simulink model "generic_IVS"  (R2024a)
settings: Solver=FixedStepDiscrete  StartTime=0.0  StopTime=inf  FixedStep=0.001  RelTol=1e-3
undefined symbols (not defined in the file): do_waypoints_tail_shifted_2, pathXY, route1_waypoint, route1_waypoint_raw, route2_waypoint, route2_waypoint_raw, route3_waypoint, route3_waypoint_raw, waypoints2
libraries: CarMaker4SL x431, slpidlib x19, dspsigops x3, simulink x1
(part 12 of 15)

== matlab function generic_IVS/CarMaker/Subsystem/Final Project1/Scenario 1/Enabled Subsystem2/MATLAB Function3 ==
  settings: updateMethod=DISCRETE  sampleTime=0.05
  data: map_boundary input; mapMatrix output size=[1000, 1000]; traffic_info input
%% ======== generate_map_ ======== Ver 2025-05-17 10:40
function mapMatrix  = generate_map_(map_boundary, traffic_info)
    %변수설정
    resolution = 0.05;
    traffic_info_mat = reshape(traffic_info(1:5*21), 5, []).';
    x_values = map_boundary(1:2:end);
    y_values = map_boundary(2:2:end);
    N = size(traffic_info_mat,1);
    x_min = min(x_values);  x_max = max(x_values);
    y_min = min(y_values);  y_max = max(y_values);
    x_size = ceil((x_max-x_min)/resolution);
    y_size = ceil((y_max-y_min)/resolution);
    
    
    mapMatrix = zeros(y_size, x_size); %출력코드
    
    for i = 1:N
        x_c = traffic_info_mat(i, 1);
        y_c = traffic_info_mat(i, 2);
        yaw = traffic_info_mat(i, 3);
        length = traffic_info_mat(i, 4);
        width = traffic_info_mat(i, 5);
        
        if yaw == -1.57079628
            yaw = -pi/2;
        elseif yaw == 1.57079628
            yaw = pi/2;
        end

        dx = length/2;  dy = width/2;
        local = [-dx,-dy; dx,-dy; dx,dy; -dx,dy];
        R = [cos(yaw), -sin(yaw); sin(yaw), cos(yaw)];
        rotated = (R*local')';
        forward_vec = [cos(yaw), sin(yaw)];
        side_vec    = [-sin(yaw), cos(yaw)];
        if yaw == -pi/2
            center = [x_c, y_c] + (length/2)*forward_vec + (width/2)*side_vec;
        else
            center = [x_c, y_c] + (length/2)*forward_vec - (width/2)*side_vec;
        end
        corners = rotated + center;
        x_idx = (corners(:,1)-x_min)/resolution + 1;
        y_idx = (y_max-corners(:,2))/resolution + 1;
        mask = poly2mask(x_idx, y_idx, y_size, x_size);
        mapMatrix(mask) = 1;
    end
end

== matlab function generic_IVS/CarMaker/Subsystem/Final Project1/Scenario 1/Enabled Subsystem2/MATLAB Function4 ==
  settings: updateMethod=DISCRETE  sampleTime=0.05
  data: map input; x_path output; startPose input; goalPose input; y_path output; mapboundary input
function [x_path, y_path] = rrt_star_planner(map, startPose, goalPose, mapboundary)
    %% ===== Persistent 저장 =====
    persistent path_initialized x_path_cached y_path_cached nPath_cached
    maxPathLength = 500;
    resolution = 0.05;

    if isempty(path_initialized)
        path_initialized = false;
        x_path_cached = zeros(maxPathLength, 1);
        y_path_cached = zeros(maxPathLength, 1);
        nPath_cached = 1;
    end

    if path_initialized
        x_path = x_path_cached(1:nPath_cached);
        y_path = y_path_cached(1:nPath_cached);
        return;
    end

    %% 설정
    visualize      = false;
    maxIter        = 5000;
    stepSize       = 2;
    goalSampleRate = 0.1;
    successDistTh  = 5;
    collisionRes   = 0.5;
    searchRadius   = 10;
    safetyDist     = 35;
    
    %% 바운더리 기반 인덱스 변환용 파라미터
    x_values = mapboundary(1:2:end);
    y_values = mapboundary(2:2:end);
    x_min = min(x_values);
    y_max = max(y_values);

    %% 실좌표 → 인덱스 변환
    toGrid = @(x, y) [(x - x_min)/resolution +  1, (y_max - y)/resolution + 1];

    start_grid = toGrid(startPose(1), startPose(2));
    goal_grid  = toGrid(goalPose(1), goalPose(2));

    %% 트리 초기화 (모든 노드는 인덱스 좌표로 유지)
    nodes = struct('x', start_grid(1), 'y', start_grid(2), ...
                   'parent', 0, 'cost', 0);

    %% 경로 및 출력 초기화
    path   = struct('x', {}, 'y', {}, 'parent', {}, 'cost', {});
    x_path = zeros(maxPathLength, 1);
    y_path = zeros(maxPathLength, 1);

    %% RRT* 메인 루프 (모든 연산 인덱스 기반)
    for iter = 1:maxIter
        if rand < goalSampleRate
            xr = goal_grid;
        else
            xr = [randi([1, size(map,2)]), randi([1, size(map,1)])];
        end

        [nearestIdx, nearXY] = findNearest(nodes, xr);
        theta = atan2(xr(2)-nearXY(2), xr(1)-nearXY(1));
        newXY = nearXY + stepSize * [cos(theta), sin(theta)];

        if isCollision(newXY, map) || ...
           isPathCollision(nearXY, newXY, map, collisionRes) || ...
           isNearObstacle(newXY, map, safetyDist)
            continue;
        end

        nearIdxs = findNearNodes(nodes, newXY, searchRadius);
        minCost   = nodes(nearestIdx).cost + norm(newXY - nearXY);
        minParent = nearestIdx;

        for idx = 1:numel(nearIdxs)
            iNode = nearIdxs(idx);
            pxy   = [nodes(iNode).x, nodes(iNode).y];
            if ~isPathCollision(pxy, newXY, map, collisionRes)
                c = nodes(iNode).cost + norm(newXY - pxy);
                if c < minCost
                    minCost   = c;
                    minParent = iNode;
                end
            end
        end

        newNode = struct('x', newXY(1), 'y', newXY(2), ...
                         'parent', minParent, 'cost', minCost);
        nodes(end+1) = newNode;
        newIdx       = numel(nodes);

        for idx = 1:numel(nearIdxs)
            iNode = nearIdxs(idx);
            pxy   = [nodes(iNode).x, nodes(iNode).y];
            c     = newNode.cost + norm([newNode.x, newNode.y] - pxy);
            if c < nodes(iNode).cost && ...
               ~isPathCollision([newNode.x,newNode.y], pxy, map, collisionRes)
                nodes(iNode).parent = newIdx;
                nodes(iNode).cost   = c;
            end
        end

        if visualize
            plot([nodes(newNode.parent).x, newNode.x], ...
                 [nodes(newNode.parent).y, newNode.y], '-r');
            hold on;
        end

        if norm(newXY - goal_grid) < successDistTh
            if visualize, disp('[-] GOAL REACHED'); end
            path = backtrace(nodes, newIdx);
            break;
        end
    end

    %% 결과 경로 반환 (인덱스 → 실좌표로 역변환)
    nPath = min(numel(path), maxPathLength);
    x_path_cached = zeros(maxPathLength, 1);
    y_path_cached = zeros(maxPathLength, 1);
    for k = 1:nPath
        x_path_cached(k) = (path(k).x - 1) * resolution + x_min;
        y_path_cached(k) = y_max - (path(k).y - 1) * resolution;
    end

    nPath_cached = nPath;
    path_initialized = true;

    %% === Lightweight Smoothing for Simulink Compatibility ===
    smooth_window = 15;  % 홀수 추천
    if nPath >= smooth_window
        x = x_path_cached(1:nPath);
        y = y_path_cached(1:nPath);

        x_smooth = movmean(x, smooth_window);
        y_smooth = movmean(y, smooth_window);

        % 재샘플링 (고정된 개수로)
        smoothN = 100;
        idx_original = linspace(1, numel(x_smooth), smoothN);
        x_path = interp1(1:numel(x_smooth), x_smooth, idx_original, 'linear')';
        y_path = interp1(1:numel(y_smooth), y_smooth, idx_original, 'linear')';
    else
        x_path = x_path_cached(1:nPath);
        y_path = y_path_cached(1:nPath);
    end


end

%% ======= 서브 함수들 =======

function [idx, xy] = findNearest(nodes, sampleXY)
    d = arrayfun(@(n) hypot(n.x - sampleXY(1), n.y - sampleXY(2)), nodes);
    [~, idx] = min(d);
    xy = [nodes(idx).x, nodes(idx).y];
end

function nearIdxs = findNearNodes(nodes, pos, radius)
    maxNodes = 1000;
    nearIdxs = zeros(1, maxNodes);
    count = 0;
    for i = 1:numel(nodes)
        if hypot(nodes(i).x - pos(1), nodes(i).y - pos(2)) <= radius
            count = count + 1;
            nearIdxs(count) = i;
        end
    end
    nearIdxs = nearIdxs(1:count);
end

function flag = isCollision(pt, map)
    x = round(pt(1)); y = round(pt(2));
    flag = x < 1 || x > size(map,2) || y < 1 || y > size(map,1) || map(y,x) == 1;
end

function flag = isPathCollision(p1, p2, map, step)
    dist = norm(p2 - p1);
    N = max(1, ceil(dist / step));
    flag = false;
    for i = 0:N
        pt = p1 + (p2 - p1) * (i / N);
        if isCollision(pt, map)
            flag = true; return;
        end
    end
end

function flag = isNearObstacle(pt, map, safeDist)
    x0 = round(pt(1)); y0 = round(pt(2));
    r  = ceil(safeDist);
    [X, Y] = meshgrid((x0 - r):(x0 + r), (y0 - r):(y0 + r));
    D2 = (X - pt(1)).^2 + (Y - pt(2)).^2;
    mask = D2 <= safeDist^2;
    X = X(mask); Y = Y(mask);
    valid = X >= 1 & X <= size(map,2) & Y >= 1 & Y <= size(map,1);
    flag  = any(map(sub2ind(size(map), Y(valid), X(valid))) == 1);
end

function path = backtrace(nodes, idx)
    maxPathLen = 500;
    dummyNode = struct('x', 0, 'y', 0, 'parent', 0, 'cost', 0);
    path = repmat(dummyNode, maxPathLen, 1);
    count = 0;
    while idx ~= 0 && count < maxPathLen
        count = count + 1;
        path(count) = nodes(idx);
        idx = nodes(idx).parent;
    end
    path = path(count:-1:1);
end

== matlab function generic_IVS/CarMaker/Subsystem/Final Project1/Scenario 1/Enabled Subsystem2/MATLAB Function ==
  settings: updateMethod=DISCRETE  sampleTime=0.05
  data: waypoints_x input; waypoints_y input; X_ego input; steering_angle output; speed output; Y_ego input; head input; goal_pose input; x_local output; y_local output
function [steering_angle, speed, x_local, y_local] = ...
    global_to_local_waypoints(waypoints_x, waypoints_y, ...
                              X_ego, Y_ego, head, goal_pose)
%#codegen

    %% 1) 파라미터
    stop_threshold          = 4.0;
    heading_align_threshold = 10.0;
    v_base                  = 5.0;   % [m/s]
    v_min                   = 1.5;
    v_max                   = 10.0;
    smooth_window           = 5;     % 웨이포인트 이동평균 윈도우
    alpha_filter            = 0.7;   % 조향각 저역통과 계수 (0~1)

    %% 2) 초기화
    x_local = 0;  y_local = 0;
    steering_angle = 0;
    speed = v_base;

    %% 3) 목표점까지 거리 계산
    goal_dist = norm([X_ego - goal_pose(1), Y_ego - goal_pose(2)]);
    if goal_dist < stop_threshold
        speed = 0; steering_angle = 0; return;
    elseif goal_dist < heading_align_threshold
        heading_error   = wrapToPi(pi/2 - head);
        steering_angle = atan2(2*2.9*sin(heading_error), goal_dist + 1e-3); %원래 1e-3
        speed           = 3;
        return;
    end

    %% 4) 유효 웨이포인트 추출 및 스무딩
    valid = ~isnan(waypoints_x) & ~isnan(waypoints_y);
    x_wp0 = waypoints_x(valid);
    y_wp0 = waypoints_y(valid);
    if numel(x_wp0)<2
        speed = 0; return;
    end
    % — 이동평균 스무딩 —
    x_wp = smoothdata(x_wp0, 'movmean', smooth_window);
    y_wp = smoothdata(y_wp0, 'movmean', smooth_window);

    %% 5) 가장 가까운 포인트 로컬 좌표
    dists = hypot(x_wp - X_ego, y_wp - Y_ego);
    [~, idx_closest] = min(dists);
    dx = x_wp(idx_closest) - X_ego;
    dy = y_wp(idx_closest) - Y_ego;
    x_local = dx*cos(-head) - dy*sin(-head);
    y_local = dx*sin(-head) + dy*cos(-head);

    %% 6) Pure Pursuit 조향각 계산
    [steer_pp, ~] = pure_pursuit(x_wp, y_wp, [X_ego, Y_ego], head);

    %% 7) 조향각 저역통과 필터
    persistent last_steer
    if isempty(last_steer)
        last_steer = steer_pp;
    end
    steering_angle = alpha_filter * last_steer + (1-alpha_filter) * steer_pp;
    last_steer = steering_angle;

    %% 8) 속도 제한
    speed = max(v_min, min(v_max, v_base));
end

%% ===== Pure Pursuit 함수 (변경 없음) =====
function [steering_angle, start_idx] = pure_pursuit(waypoints_x, waypoints_y, vehicle_position, head)
    persistent last_target_idx;
    if isempty(last_target_idx), last_target_idx = 1; end

    WHEEL_BASE = 20.0;
    lookahead_dist = 5.5;
    num_points = length(waypoints_x);

    x_ego = vehicle_position(1);
    y_ego = vehicle_position(2);
    local_waypoints = zeros(num_points, 2);

    for i = 1:num_points
        dx = waypoints_x(i) - x_ego;
        dy = waypoints_y(i) - y_ego;
        local_waypoints(i,:) = [ dx*cos(-head)-dy*sin(-head), ...
                                 dx*sin(-head)+dy*cos(-head) ];
    end

    d2 = hypot(waypoints_x - x_ego, waypoints_y - y_ego);
    [~, closest_idx] = min(d2);
    start_idx = max(last_target_idx, closest_idx);

    target_idx = -1;
    for i = start_idx:num_points
        if norm(local_waypoints(i,:))>lookahead_dist && local_waypoints(i,1)>0
            target_idx = i; break;
        end
    end
    if target_idx<0
        for i = 1:start_idx-1
            if norm(local_waypoints(i,:))>lookahead_dist && local_waypoints(i,1)>0
                target_idx = i; break;
            end
        end
    end
    if target_idx<0
        steering_angle = 0; return;
    end

    pt = local_waypoints(target_idx,:);
    alpha = wrapToPi(atan2(pt(2),pt(1)));
    ld = min(max(norm(pt),2.0),20.0);
    steering_angle = atan2(2*WHEEL_BASE*sin(alpha), ld);

    last_target_idx = target_idx;
end

%% ===== 각도 wrap 함수 (변경 없음) =====
function angle = wrapToPi(theta)
    angle = mod(theta + pi, 2*pi) - pi;
end

== matlab function generic_IVS/CarMaker/Subsystem/Final Project/Scenario 1/MATLAB Function ==
  settings: updateMethod=DISCRETE  sampleTime=1
  data: waypoints_x input; waypoints_y input; X_ego input; Y_ego input; head input; steering_angle output; goal_pose input; speed output
function [steering_angle, speed] = ...
    global_to_local_waypoints(waypoints_x, waypoints_y, ...
                              X_ego, Y_ego, head, goal_pose)
%#codegen
% 글로벌 웨이포인트 → 로컬 좌표 변환 + 조향각 계산 (Pure Pursuit)
% 후방 포인트는 무시하며, 초기에는 아무 유효 포인트 없을 수 있음

    %% 파라미터
    L = 4.0;               % 휠베이스
    epsilon = 1e-3;        % 안정화용
    lookahead_dist = 1.0;  % 추적 기준 거리
    stop_threshold = 2.8;  % 완전 정지 거리
    heading_align_threshold = 15.0;  % 헤딩 조정 시작 거리

    %% 초기값 설정 (모든 실행 경로 보장)
    local_point = [0 0];
    dist = 0;
    idx_closest = 1;
    steering_angle = 0;
    goal_dist = norm([X_ego - goal_pose(1), Y_ego - goal_pose(2)]);
    
    %% 정지 조건
    if goal_dist < stop_threshold
        speed = 0;
        steering_angle = 0;
        return;
    end

    %% 헤딩 정렬 조건 적용
    if goal_dist < heading_align_threshold
        heading_error = wrapToPi(pi/2 - head);  % 90도 방향으로 정렬
        steering_angle = atan2(2 * L * sin(heading_error), goal_dist + epsilon);
        speed = 0;
        % 이 부분에서 
        return;
    end

    %% 1) NaN 제거
    valid_idx = ~isnan(waypoints_x) & ~isnan(waypoints_y);
    x_wp = waypoints_x(valid_idx);
    y_wp = waypoints_y(valid_idx);
    N = numel(x_wp);

    if N == 0
        speed = 0;
        return;
    end

    %% 2) 차량 기준 상대 위치 계산
    dx_all = x_wp(:)' - X_ego;
    dy_all = y_wp(:)' - Y_ego;

    %% 3) 차량 전방 필터
    forward_vec = [cos(head); sin(head)];
    rel_pos = [dx_all; dy_all];
    dot_products = forward_vec' * rel_pos;
    is_in_front = dot_products > 0;

    %% 4) 전방 포인트가 없다면: 정지 상태 유지
    if ~any(is_in_front)
        speed = 0;
        return;
    end

    %% 5) 가장 가까운 전방 인덱스 찾기
    d2_all = dx_all.^2 + dy_all.^2;
    d2_all(~is_in_front) = Inf;
    [~, idx_closest] = min(d2_all);

    %% 6) 전체 로컬 좌표 변환
    c = cos(-head); s = sin(-head);
    R = [c, -s; s, c];
    rel_global = [x_wp - X_ego, y_wp - Y_ego]';
    local_wp = R * rel_global;       % 2×N
    Local_Waypoints = local_wp';     % Nx2
    local_point = Local_Waypoints(idx_closest, :);
    dist = sqrt(d2_all(idx_closest));

    %% 7) 추적 포인트 찾기 (lookahead 거리 기준)
    target_idx = idx_closest;
    for i = idx_closest+1:N
        d = norm(Local_Waypoints(i,:) - Local_Waypoints(idx_closest,:));
        if d > lookahead_dist
            target_idx = i;
            break;
        end
    end

    %% 8) 조향각 계산 (Pure Pursuit)
    x_t = Local_Waypoints(target_idx, 1);
    y_t = Local_Waypoints(target_idx, 2);
    L_d = sqrt(x_t^2 + y_t^2 + epsilon);
    alpha = atan2(y_t, x_t);
    steering_angle = atan2(2 * L * sin(alpha), L_d);

    %% 9) 속도 설정
    speed = 10;
end

%% ===== 각도 wrap =====
function angle = wrapToPi(theta)
    angle = mod(theta + pi, 2*pi) - pi;
end

== matlab function generic_IVS/CarMaker/Subsystem/Final Project1/Scenario 1/MATLAB Function15 ==
  settings: updateMethod=DISCRETE  sampleTime=0.05
  data: ego_pos input; ego_yaw input; ego_vx input; ego_lane_idx input; traffic_info input; target_speed output; traffic_lane_idx input; debug_time_gap output; gate_flag input
function [target_speed, debug_time_gap] = acc_timegap_based( ...
    ego_pos, ego_yaw, ego_vx, ego_lane_idx, ...
    traffic_info, traffic_lane_idx, gate_flag)

    % 기본 설정
    default_speed = 15.0;      % m/s (기본 크루즈 속도)
    safe_gap_time = 2.5;       % 안전 시간 간격 (초)
    emergency_gap_time = 1.8;  % 비상 시간 간격 (초)

    % 이전 속도 유지용 변수
    persistent last_speed
    if isempty(last_speed)
        last_speed = default_speed;
    end

    % 전방 차량 정보 분리
    traffic_pos = traffic_info(:, 1:2);   % 위치 [8x2]
    traffic_vx = traffic_info(:, 3);      % 속도 [8x1]
    L = size(traffic_info, 1);            % 차량 수

    % 초기값 설정
    min_gap_time = inf;
    front_vx = 0;
    found = false;

    ego_dir = [cos(ego_yaw); sin(ego_yaw)];  % 주행 방향 단위 벡터

    for i = 1:L
        if traffic_lane_idx(i) == ego_lane_idx
            dx = traffic_pos(i,1) - ego_pos(1);
            dy = traffic_pos(i,2) - ego_pos(2);
            rel_vec = [dx; dy];

            if dot(rel_vec, ego_dir) > 0  % 전방 차량인지 확인
                dist = norm(rel_vec);

                % ego 속도가 0이면 분모 0 방지
                if ego_vx > 0
                    time_gap = dist / ego_vx;
                else
                    time_gap = inf;
                end

                if time_gap < min_gap_time
                    min_gap_time = time_gap;
                    front_vx = traffic_vx(i);
                    found = true;
                end
            end
        end
    end

    % 기본 속도 계산 (gate_flag 고려 없이)
    speed = default_speed;
    if found
        if min_gap_time < emergency_gap_time
            speed = 0;  % 매우 위험 → 정지
        elseif min_gap_time < safe_gap_time
            ratio = (min_gap_time - emergency_gap_time) / (safe_gap_time - emergency_gap_time);
            speed = front_vx * ratio;
        end
    end

    % gate_flag에 따라 속도 조정
    if gate_flag
        last_speed = speed * 0.5;  % 속도 절반으로 줄이기
    else
        last_speed = speed;        % 원래 속도 복구
    end

    target_speed = last_speed;

    % 디버깅 정보 출력용
    debug_time_gap = min_gap_time;

%% 
%% 


    persistent prev_x
    if isempty(prev_x)
        prev_x = ego_pos(1);
    end

    x_min = -160;
    x_max = 30;
    v_zone = 30;

    curr_x = ego_pos(1);

    % x증가방향 및 구간내 판정
    if curr_x >= x_min && curr_x <= x_max && (curr_x - prev_x) > 0
        target_speed = v_zone;
    % else
        % v_target = nan;   % 구간밖 or 반대방향: 무시
    end

    prev_x = curr_x;    % 이전값 업데이트
end


% function [target_speed, debug_time_gap] = acc_timegap_based( ...
%     ego_pos, ego_yaw, ego_vx, ego_lane_idx, ...
%     traffic_info, traffic_lane_idx, gate_flag)
% 
% 
%     % 기본 설정
%     default_speed = 15.0;      % m/s (기본 크루즈 속도)
%     safe_gap_time = 2.5;       % 안전 시간 간격 (초)
%     emergency_gap_time = 1.8;  % 비상 시간 간격 (초)
% 
%     % 전방 차량 정보 분리
%     traffic_pos = traffic_info(:, 1:2);   % 위치 [8x2]
%     traffic_vx = traffic_info(:, 3);      % 속도 [8x1]
%     L = size(traffic_info, 1);            % 차량 수
% 
%     % 초기값 설정
%     min_gap_time = inf;
%     front_vx = 0;
%     found = false;
% 
%     ego_dir = [cos(ego_yaw); sin(ego_yaw)];  % 주행 방향 단위 벡터
% 
%     for i = 1:L
%         if traffic_lane_idx(i) == ego_lane_idx
%             dx = traffic_pos(i,1) - ego_pos(1);
%             dy = traffic_pos(i,2) - ego_pos(2);
%             rel_vec = [dx; dy];
% 
%             if dot(rel_vec, ego_dir) > 0  % 전방 차량인지 확인
%                 dist = norm(rel_vec);
% 
%                 % ego 속도가 0이면 분모 0 방지
%                 if ego_vx > 0
%                     time_gap = dist / ego_vx;
%                 else
%                     time_gap = inf;
%                 end
% 
%                 if time_gap < min_gap_time
%                     min_gap_time = time_gap;
%                     front_vx = traffic_vx(i);
%                     found = true;
%                 end
%             end
%         end
%     end
% 
%     % 속도 결정 로직
%     target_speed = default_speed;
% 
%     if found
%         if min_gap_time < emergency_gap_time
%             target_speed = 0;  % 매우 위험 → 정지
%         elseif min_gap_time < safe_gap_time
%             ratio = (min_gap_time - emergency_gap_time) / (safe_gap_time - emergency_gap_time);
%             target_speed = front_vx * ratio;
%         else
%             target_speed = default_speed;
%         end
%     end
% 
%     if gate_flag ==1
% 
%     % 디버깅 정보 출력용
%     debug_time_gap = min_gap_time;
% end
% 
%

== matlab function generic_IVS/CarMaker/Subsystem/Final Project1/Scenario 1/MATLAB Function16 ==
  settings: updateMethod=DISCRETE  sampleTime=0.05
  data: s_ref input; global_path output; global_waypoint_2 input; Ego_x input; Ego_y input; Ego_Yaw input; Ego_Vx input; Ego_Ax input; target_speed input; obs_pre input; TargetTolgateLane input; gate_flag input
function global_path  = trajectory_path(s_ref, global_waypoint_2, Ego_x, Ego_y, Ego_Yaw, Ego_Vx, Ego_Ax, target_speed, obs_pre, TargetTolgateLane, gate_flag)
    LANE_WIDTH = 3.0;
    CENTER_LANE = 2;
    TargetTolgateLane_d = (TargetTolgateLane - CENTER_LANE) * LANE_WIDTH;



    mapx= global_waypoint_2(:,1);
    mapy= global_waypoint_2(:,2);
    
    % === 초기 자차 위치 및 상태 === %
    % traffic_info: [8 x 10] → 각 행: [x, y, vx, vy, ax, ay, yaw, yawRate, length, width]
    obs=obs_pre(:,[1:8]);

    x0 = Ego_x; %
    y0 = Ego_y; %
    yaw0 = Ego_Yaw; % 
    v0 = Ego_Vx; a0 = Ego_Ax; %% 초기값 

    % 1. Frenet 좌표계 위치 (s0, d0) 계산
    [s0, d0] = get_frenet(x0, y0, mapx, mapy);

    % 2. 기준 경로에서의 진행 방향 (yaw_path) 계산
    [~, ~, yaw_path] = get_cartesian(s0, d0, mapx, mapy, s_ref);

    % 3. 경로 기준 상대 진행 방향 계산
    yawi = yaw0 - yaw_path;

    % 4. Frenet 상태 초기값
    si    = s0;
    si_d  = v0 * cos(yawi);
    si_dd = a0 * cos(yawi);
    sf_d  = target_speed; %%%%%%%%%%%%%%%%%%%%%%%%%%%%%%%%%%%%%%%%%%%
    sf_dd = 0;

    di    = d0;
    di_d  = v0 * sin(yawi);
    di_dd = a0 * sin(yawi);
    df_d  = 0;
    df_dd = 0;

    opt_d = di;  % 횡 방향 목표 유지
    
    %% 
   
    [path, opt_ind] = frenet_optimal_planning(...
                                              si, si_d, si_dd, sf_d, sf_dd, di, di_d, di_dd, ...
                                              df_d, df_dd, obs, mapx, mapy, s_ref, opt_d, gate_flag, TargetTolgateLane_d); %%%%%%%%%%%%%%%%%%%%%%%%%%%%%%%%obs 만처리하면됨 
   
    %% 출력
    global_path = [path(opt_ind).x(1:path(opt_ind).len)', path(opt_ind).y(1:path(opt_ind).len)'];  % N×2
    
    
    % 
    % % === 디버깅용 시각화 ===
    % figure(1); clf; hold on; axis equal;
    % plot(mapx, mapy, 'k--'); % 기준 경로
    % plot(global_path(:,1), global_path(:,2), 'b-', 'LineWidth', 2); % 최적 궤적
    % plot(Ego_x, Ego_y, 'ro'); % 자차 현재 위치
    % title('Selected Optimal Trajectory');
    % grid on;

    
end

function [path, opt_ind] = frenet_optimal_planning(...
                                                  si, si_d, si_dd, sf_d, sf_dd, di, di_d, di_dd, ...
                                                  df_d, df_dd, obs, mapx, mapy, s_ref, opt_d, gate_flag, TargetTolgateLane_d)
    % 1. Frenet 궤적 후보 생성
    [fplist, MAX_len, LENG_path] = calc_frenet_paths(...
                                                    si, si_d, si_dd, sf_d, sf_dd, di, di_d, di_dd, ...
                                                    df_d, df_dd, opt_d, gate_flag, TargetTolgateLane_d);


    % 2. Global 궤적 변환
    fplist = calc_global_paths(fplist, mapx, mapy, s_ref);

    % 3. 제약조건 및 충돌 검사 → 유효 trajectory만 반환
    [valid_paths, num_valid] = check_path(fplist, obs, MAX_len, LENG_path);

    % 4. 최적 경로 선택
    min_cost = inf;
    opt_ind = 1;  % 초기값

    for i = 1:num_valid
        if valid_paths(i).c_tot < min_cost
            min_cost = valid_paths(i).c_tot;
            opt_ind = i;
        end
    end

    % 5. 출력 (최종 유효 경로들)
    path = valid_paths;
end

    

function [fplist, MAX_len, LENG_path] = calc_frenet_paths(...
                                                            si, si_d, si_dd, sf_d, sf_dd, di, di_d, di_dd, ...
                                                            df_d, df_dd, opt_d, gate_flag, TargetTolgateLane_d)
  
    % % 차선 번호(1,2,3)를 실제 Frenet d 좌표로 변환
    % LANE_WIDTH = 3;     % 실제 차선 폭 [m]
    % CENTER_LANE = 2;      % 중앙 차선 번호
    % TargetTolgateLane_d = (TargetTolgateLane - CENTER_LANE) * LANE_WIDTH;


    
    TARGET_SPEED = sf_d;
    DF_SET = linspace(-3, 3, 3); 
    DT = 0.05; 
    DT_T = 0.2; 
    MIN_T = 2; 
    MAX_T = 4; 
     % K_J Jerk 웨이트 s,d 둘다 , K_T t_f에 대한 항, K_D Diff d에대한 diff, K_V s에 대한 diff(속도 s_d에 대한 diff)
    MAX_len= (MAX_T/DT)+1;

    K_J = 0.1; K_T = 1; K_D = 1; K_V = 1;

    W_LAT = 1.0; W_LON = 1.0; %종방향 횡방향 웨이트
    
    LENG_path = 3*(MAX_T-MIN_T)/DT_T; 
    fp_templet = struct( ...
    't', zeros(1,MAX_len), ...
    'd', zeros(1,MAX_len), 'd_d', zeros(1,MAX_len), 'd_dd', zeros(1,MAX_len), 'd_ddd', zeros(1,MAX_len), ...
    's', zeros(1,MAX_len), 's_d', zeros(1,MAX_len), 's_dd', zeros(1,MAX_len), 's_ddd', zeros(1,MAX_len), ...
    'c_lat', 0, 'c_lon', 0, 'c_tot', 0, ...
    'x', zeros(1,MAX_len), 'y', zeros(1,MAX_len), 'yaw', zeros(1,MAX_len), ...
    'ds', zeros(1,MAX_len), 'kappa', zeros(1,MAX_len), ...
    'len', 0);

    fplist = repmat(fp_templet, 1, LENG_path);  % 빈 구조체 배열로 초기화
    index=1;
    for df = DF_SET
        for T = MIN_T:DT_T:MAX_T
            
            % Lateral trajectory (Quintic)
            [a0_d, a1_d, a2_d, a3_d, a4_d, a5_d] = calc_quintic(di, di_d, di_dd, df, df_d, df_dd, T);
            
            t = 0:DT:T;
            
            d = a0_d + a1_d*t + a2_d*t.^2 + a3_d*t.^3 + a4_d*t.^4 + a5_d*t.^5;
            d_d = a1_d + 2*a2_d*t + 3*a3_d*t.^2 + 4*a4_d*t.^3 + 5*a5_d*t.^4;
            d_dd = 2*a2_d + 6*a3_d*t + 12*a4_d*t.^2 + 20*a5_d*t.^3;
            d_ddd = 6*a3_d + 24*a4_d*t + 60*a5_d*t.^2;
            
            
            % Longitudinal trajectory (Quartic)
            %sf_d에 Target Speed를 기준으로 여러개 생성해야된다
            %sf 인자는 어디로 갔나
            [a0_s, a1_s, a2_s, a3_s, a4_s] = calc_quartic(si, si_d, si_dd, sf_d, sf_dd, T);
            s = a0_s + a1_s*t + a2_s*t.^2 + a3_s*t.^3 + a4_s*t.^4;
            s_d = a1_s + 2*a2_s*t + 3*a3_s*t.^2 + 4*a4_s*t.^3;
            s_dd = 2*a2_s + 6*a3_s*t + 12*a4_s*t.^2;
            s_ddd = 6*a3_s + 24*a4_s*t;
            
           
            %% 비용 계산
            J_lat = sum(d_ddd.^2); %적분항 인데 왜 T로 안나눠 임마 
            J_lon = sum(s_ddd.^2); %적분항 
            if gate_flag
                d_gate_weight = 10000000000;
                d_diff = (d(end) - TargetTolgateLane_d)^2 * d_gate_weight;
            else
                d_diff = (d(end) - opt_d)^2;
            end

            % if gate_flag
            %     opt_d = TargetTolgateLane_d;
            % else
            %     opt_d = di;
            % end


            s_diff = (TARGET_SPEED - s_d(end))^2; %ACC랑 최대한 유지하기 위함

            
            % if gate_flag
            %     d_gate_weight = 10000000000;
            %     d_diff = (d(end) - TargetTolgateLane_d)^2 * d_gate_weight;
            %     fprintf('[DEBUG] df = %.2f | d(end) = %.2f | target_d = %.2f | cost = %.2e\n', ...
            %             df, d(end), TargetTolgateLane_d, d_diff);
            % else
            %     d_diff = (d(end) - opt_d)^2;
            % end

            %% 비용함수
            c_lat = K_J * J_lat  + K_D * d_diff + K_T * T; %% cost_lateral
            c_lon = K_J * J_lon  + K_V * s_diff + K_T * T; %% cost_longitual
            c_tot = W_LAT * c_lat + W_LON * c_lon; %% total Cost가 낮은것을 선택

            len = length(t);  % ← 이 줄이 꼭 필요!

            % 1. fp 템플릿 기반 새 구조체 생성
            fp = fp_templet;

            % 2. 유효 길이 저장
            fp.len = len;

            % 3. 시간 및 궤적 데이터 복사
            fp.t(1:len)     = t;
            fp.d(1:len)     = d;
            fp.d_d(1:len)   = d_d;
            fp.d_dd(1:len)  = d_dd;
            fp.d_ddd(1:len) = d_ddd;

            fp.s(1:len)     = s;
            fp.s_d(1:len)   = s_d;
            fp.s_dd(1:len)  = s_dd;
            fp.s_ddd(1:len) = s_ddd;

            % 4. 비용도 할당
            fp.c_lat = c_lat;
            fp.c_lon = c_lon;
            fp.c_tot = c_tot;

            % 5. fplist에 대입
            fplist(index) = fp;
            if(index<LENG_path)
            index = index +1;
            end
        end
    end
end

function fplist = calc_global_paths(fplist, mapx, mapy, s_ref)
    for i = 1:length(fplist)
        fp = fplist(i);
        len = fp.len;

        % === Global 좌표 변환 === %
        for j = 1:len
            [fp.x(j), fp.y(j), ~] = get_cartesian(fp.s(j), fp.d(j), mapx, mapy, s_ref);
        end

        % === Yaw, ds 계산 === %
        for j = 1:len-1
            dx = fp.x(j+1) - fp.x(j);
            dy = fp.y(j+1) - fp.y(j);
            fp.yaw(j) = atan2(dy, dx);
            fp.ds(j) = hypot(dx, dy);
        end
        if len >= 2
            fp.yaw(len) = fp.yaw(len - 1);
            fp.ds(len)  = fp.ds(len - 1);
        else
            fp.yaw(len) = 0;
            fp.ds(len)  = 1e-6;  % 너무 작지 않게 보호
        end

        % === 곡률 계산 === %
        for j = 1:len-1
            dyaw = atan2(sin(fp.yaw(j+1) - fp.yaw(j)), cos(fp.yaw(j+1) - fp.yaw(j)));
            fp.kappa(j) = dyaw / fp.ds(j);
        end
        if len >= 2
            fp.kappa(len) = fp.kappa(len - 1);
        else
            fp.kappa(len) = 0;
        end

        % 업데이트된 fp 구조체 다시 저장
        fplist(i) = fp;
    end
end

function [valid_paths, numValid] = check_path(fplist, obs, MAX_len, LENG_path)
    % 정적 템플릿 구조체 선언
    fp_templet = struct( ...
        't', zeros(1,MAX_len), ...
        'd', zeros(1,MAX_len), 'd_d', zeros(1,MAX_len), 'd_dd', zeros(1,MAX_len), 'd_ddd', zeros(1,MAX_len), ...
        's', zeros(1,MAX_len), 's_d', zeros(1,MAX_len), 's_dd', zeros(1,MAX_len), 's_ddd', zeros(1,MAX_len), ...
        'c_lat', 0, 'c_lon', 0, 'c_tot', 0, ...
        'x', zeros(1,MAX_len), 'y', zeros(1,MAX_len), 'yaw', zeros(1,MAX_len), ...
        'ds', zeros(1,MAX_len), 'kappa', zeros(1,MAX_len), ...
        'len', 0);

    % 제약 조건
    V_MAX = 30;
    ACC_MAX = 5;
    K_MAX = 1.5;

    % 고정 크기 구조체 배열 선언
    valid_paths = repmat(fp_templet, 1, LENG_path);
    index = 1;
    numValid = 0;

    for i = 1:length(fplist)
        fp = fplist(i);
        len = fp.len;
        max_T = fp.t(len);
        acc_squared = fp.s_dd(1:len).^2;  % s 방향에 대한 가속도만 고려
        

        if all(fp.s_d(1:len) > V_MAX)
            parksangwoo=1;
            continue;
        elseif any(acc_squared > ACC_MAX^2)
            parksangwoo=2;
            continue;
        elseif any(abs(fp.kappa(1:len)) > K_MAX)
            parksangwoo=3;
            continue;
        elseif collision_check(fp, obs, len, max_T)
            parksangwoo=4;
            continue;
        elseif any(abs(fp.d(1:len)) > 3.9)
            parksangwoo=5;
            continue;
        else
            valid_paths(index) = fp;
            index = index + 1;
            numValid = numValid + 1;
        end
    end

end

function collision = collision_check(fp, obs, len, max_T)
    % 충돌 검사 함수 (다른 차량의 예측 경로를 고려)
    % fp: 현재 차량 경로
    % obs: 다른 차량의 정보 (초기 위치, 속도, 헤딩, 가속도 등)
    % MAX_len: 최대 길이
    % T: 예측 시간 (초)
    % dt: 시간 간격
    
    CAR_RADIUS = 2;
    OBSTACLE_RADIUS = 0.5;
    SAFE_DIST_SQ = (CAR_RADIUS + OBSTACLE_RADIUS)^2;
    
    collision = false;
    % traffic_info: [8 x 10] → 각 행: [1x, 2y, 3vx, 4vy, 5ax, 6ay, 7yaw, yawRate, length, width]
    
    % 예측 경로 계산
    for i = 1:size(obs, 1)
        % 다른 차량의 초기 위치와 속도, 헤딩, 가속도를 얻음
        x0 = obs(i, 1); % x 좌표
        y0 = obs(i, 2); % y 좌표
        v0 = obs(i, 3); % 속도
        yaw0 = obs(i, 7); % 헤딩 각도
        a0 = obs(i, 5); % 가속도
        yaw_rate= obs(i, 8);
        
        % 차량의 예측 경로를 계산
        [x_pred, y_pred] = predict_vehicle_trajectory_CTRV(x0, y0, v0, yaw0, yaw_rate, len, max_T);
        
        % 예측 경로와 현재 경로 간의 충돌 검사
        for j = 1:len
            % 현재 경로의 각 점과 예측 경로 간의 거리 계산
            dx = fp.x(j) - x_pred;
            dy = fp.y(j) - y_pred;
            dists_sq = dx.^2 + dy.^2;
            
            if any(dists_sq <= SAFE_DIST_SQ)
                collision = true;  % 충돌 발생
                return;
            end
        end
    end
end

% 
% function [x_pred, y_pred] = predict_vehicle_trajectory(x0, y0, v0, yaw0, a0, len, max_T)
%     % 차량 예측 경로 계산 (CTRV 모델)
%     % x0, y0: 초기 위치 (차량)
%     % v0: 초기 속도
%     % yaw0: 초기 헤딩 각도
%     % a0: 초기 가속도
%     % T: 예측 시간 (초)
%     % dt: 시간 간격
%     N=len-1;
%     dt = max_T/N;  % 예측 시간 동안의 단계 수 %%이거필요없는거아냐?
%     x_pred = zeros(1, len);
%     y_pred = zeros(1, len);
% 
%     for i = 1:len
%         % 속도와 가속도에 따른 위치 업데이트
%         v = v0 + a0 * i * dt;  % 일정한 가속도를 고려한 속도 업데이트
%         x_pred(i) = x0 + v * cos(yaw0) * i * dt;
%         y_pred(i) = y0 + v * sin(yaw0) * i * dt;
%     end
% end

% %
% function [x_pred, y_pred] = predict_vehicle_trajectory_CV(x0, y0, v0, yaw0, len, max_T)
%     % 차량 예측 경로 계산 (CV 모델)
%     % x0, y0: 초기 위치 (차량)
%     % v0: 초기 속도
%     % yaw0: 초기 헤딩 각도
%     % len: 예측 길이
%     % max_T: 예측 시간 (초)
% 
%     N = len - 1;  % 예측 단계 수
%     dt = max_T / N;  % 시간 간격
% 
%     % 예측된 위치 저장 변수
%     x_pred = zeros(1, len);
%     y_pred = zeros(1, len);
% 
%     for i = 1:len
%         % 일정한 속도를 고려한 위치 업데이트
%         x_pred(i) = x0 + v0 * cos(yaw0) * i * dt;  % x 좌표
%         y_pred(i) = y0 + v0 * sin(yaw0) * i * dt;  % y 좌표
%     end
% end

% function [x_pred, y_pred, yaw_pred] = predict_vehicle_trajectory_CTRA(x0, y0, v0, yaw0, a0, yaw_rate, len, max_T)
%     % 차량 예측 경로 계산 (CTRA 모델)
%     % x0, y0: 초기 위치 (차량)
%     % v0: 초기 속도
%     % yaw0: 초기 헤딩 각도
%     % a0: 초기 가속도
%     % yaw_rate: 일정한 회전 각속도
%     % len: 예측 시간 단계 수
%     % max_T: 예측 시간 (초)
% 
%     N = len - 1;  % 예측 단계 수
%     dt = max_T / N;  % 시간 간격
% 
%     % 예측된 위치와 헤딩 각도 저장 변수
%     x_pred = zeros(1, len);
%     y_pred = zeros(1, len);
%     yaw_pred = zeros(1, len);
% 
%     for i = 1:len
%         % 속도와 가속도에 따른 위치 업데이트
%         v = v0 + a0 * i * dt;  % 일정한 가속도를 고려한 속도 업데이트
%         x_pred(i) = x0 + v * cos(yaw0 + yaw_rate * i * dt) * i * dt;
%         y_pred(i) = y0 + v * sin(yaw0 + yaw_rate * i * dt) * i * dt;
%         yaw_pred(i) = yaw0 + yaw_rate * i * dt;  % 회전 각도 업데이트
%     end
% end

function [x_pred, y_pred, yaw_pred] = predict_vehicle_trajectory_CTRV(x0, y0, v0, yaw0, yaw_rate, len, max_T)
    % 차량 예측 경로 계산 (CTRV 모델)
    % x0, y0: 초기 위치 (차량)
    % v0: 초기 속도
    % yaw0: 초기 헤딩 각도
    % yaw_rate: 일정한 회전 각속도
    % len: 예측 시간 단계 수
    % max_T: 예측 시간 (초)
    
    N = len - 1;  % 예측 단계 수
    dt = max_T / N;  % 시간 간격
    
    % 예측된 위치와 헤딩 각도 저장 변수
    x_pred = zeros(1, len);
    y_pred = zeros(1, len);
    yaw_pred = zeros(1, len);
    
    for i = 1:len
        % 일정한 속도와 회전 각속도를 고려하여 위치 업데이트
        % v0는 일정하므로 위치 업데이트에 반영
        x_pred(i) = x0 + v0 * (sin(yaw0 + yaw_rate * i * dt) - sin(yaw0)) / yaw_rate;
        y_pred(i) = y0 + v0 * (-cos(yaw0 + yaw_rate * i * dt) + cos(yaw0)) / yaw_rate;
        yaw_pred(i) = yaw0 + yaw_rate * i * dt;  % 회전 각도 업데이트
    end
end


% function collision = collision_check(fp, obs_global)
%     CAR_RADIUS = 2;
%     OBSTACLE_RADIUS = 0.5;
%     SAFE_DIST_SQ = (CAR_RADIUS + OBSTACLE_RADIUS)^2;
% 
%     len = fp.len;
%     collision = false;
% 
%     for i = 1:size(obs_global, 1)
%         dx = fp.x(1:len) - obs_global(i,1);
%         dy = fp.y(1:len) - obs_global(i,2);
%         dists_sq = dx.^2 + dy.^2;
% 
%         if any(dists_sq <= SAFE_DIST_SQ)
%             collision = true;
%             return;
%         end
%     end
% end



function [s, d] = get_frenet(x, y, x_ref, y_ref)
    idx = get_closest_waypoint(x, y, x_ref, y_ref);
    if idx == 1
        prev_idx = 1; next_idx = 2;
    elseif idx == length(x_ref)
        prev_idx = length(x_ref) - 1; next_idx = length(x_ref);
    else
        prev_idx = idx - 1; next_idx = idx;
    end
    vec_path = [x_ref(next_idx) - x_ref(prev_idx); y_ref(next_idx) - y_ref(prev_idx)];
    vec_ego  = [x - x_ref(prev_idx); y - y_ref(prev_idx)];
    proj = dot(vec_path, vec_ego) / norm(vec_path)^2 * vec_path;
    perp = vec_ego - proj;
    d = norm(perp);
    if det([vec_path, vec_ego]) < 0
        d = -d;
    end
    s = 0;
    for i = 1:(prev_idx - 1)
        s = s + norm([x_ref(i+1) - x_ref(i), y_ref(i+1) - y_ref(i)]);
    end
    s = s + norm(proj);
end

function [x, y, heading] = get_cartesian(s, d, x_ref, y_ref, s_ref)
    s = mod(s, s_ref(end));
    idx = find(s_ref <= s, 1, 'last');
    if idx >= length(s_ref), idx = length(s_ref) - 1; end
    dx = x_ref(idx+1) - x_ref(idx);
    dy = y_ref(idx+1) - y_ref(idx);
    heading = atan2(dy, dx);
    ds = s - s_ref(idx);
    x_base = x_ref(idx) + ds * cos(heading);
    y_base = y_ref(idx) + ds * sin(heading);
    x = x_base + d * cos(heading + pi/2);
    y = y_base + d * sin(heading + pi/2);
end

function idx = get_closest_waypoint(x, y, x_ref, y_ref)
    dists = sqrt((x_ref - x).^2 + (y_ref - y).^2);
    [~, idx] = min(dists);
end

function [a0, a1, a2, a3, a4, a5] = calc_quintic(xi, vi, ai, xf, vf, af, T)
    a0 = xi;
    a1 = vi;
    a2 = 0.5 * ai;
    A = [T^3, T^4, T^5;
         3*T^2, 4*T^3, 5*T^4;
         6*T, 12*T^2, 20*T^3];
    b = [xf - a0 - a1*T - a2*T^2;
         vf - a1 - 2*a2*T;
         af - 2*a2];
    x = A\b;
    a3 = x(1); a4 = x(2); a5 = x(3);
end

function [a0, a1, a2, a3, a4] = calc_quartic(xi, vi, ai, vf, af, T)
    a0 = xi;
    a1 = vi;
    a2 = 0.5 * ai;
    A = [3*T^2, 4*T^3;
         6*T, 12*T^2];
    b = [vf - a1 - 2*a2*T;
         af - 2*a2];
    x = A\b;
    a3 = x(1); a4 = x(2);
end

== matlab function generic_IVS/CarMaker/Subsystem/Final Project1/Scenario 1/MATLAB Function17 ==
  settings: updateMethod=DISCRETE  sampleTime=0.05
  data: poly_coeff input; lateral_error output; velocity input; lookahead_time input; x_lookahead output; delta_ff output; dy output; d2y output; kappa output
% function [lateral_error, x_lookahead, delta_ff, dy, d2y, kappa] = compute_lateral_error_(poly_coeff, velocity, lookahead_time)
% % ------------------------------------------------------------
% % 경로 다항식 기반 곡률 및 조향각 계산 (스무딩 포함)
% % Waypoint 부족 시 조향각 0 처리
% % ------------------------------------------------------------
% 
% % 휠베이스
% L = 2.9;
% 
% % Waypoint 부족으로 poly_coeff가 모두 0일 경우 → 계산 중단
% if all(poly_coeff == 0)
%     lateral_error = 0;
%     x_lookahead = velocity * lookahead_time;
%     delta_ff = 0;
%     dy = 0;
%     d2y = 0;
%     kappa = 0;
%     return;
% end
% 
% % 다항식 계수 추출
% a = 0; b = 0; c = 0; d = 0;
% n = length(poly_coeff);
% if n == 4
%     a = poly_coeff(1); b = poly_coeff(2); c = poly_coeff(3); d = poly_coeff(4);
% elseif n == 3
%     b = poly_coeff(1); c = poly_coeff(2); d = poly_coeff(3);
% elseif n == 2
%     c = poly_coeff(1); d = poly_coeff(2);
% else
%     d = poly_coeff(1);
% end
% 
% % 1. lateral error (x = 0)
% lateral_error = d;
% 
% % 2. lookahead 위치
% x_lookahead = velocity * lookahead_time;
% 
% % 3. dy, d2y
% dy = 3*a*x_lookahead^2 + 2*b*x_lookahead + c;
% d2y = 6*a*x_lookahead + 2*b;
% 
% % 4. kappa 계산 (수치 안정성 보장)
% denominator = (1 + dy^2)^(3/2);
% if denominator < 1e-6
%     denominator = 1e-6;
% end
% kappa = d2y / denominator;
% 
% % 5. 조향각 계산
% delta_now = L * kappa;
% 
% % 6. Moving Average Filter 적용 (스무딩)
% persistent delta_buffer
% if isempty(delta_buffer)
%     delta_buffer = zeros(1, 30);  % 최근 30개 저장
% end
% 
% % shift + 최신값 추가
% delta_buffer = [delta_now, delta_buffer(1:end-1)];
% 
% % 평균값 출력
% delta_ff = mean(delta_buffer);
% 
% end
function [lateral_error, x_lookahead, delta_ff, dy, d2y, kappa] = compute_lateral_error_(poly_coeff, velocity, lookahead_time)
% ------------------------------------------------------------
% 경로 다항식 기반 곡률 및 조향각 계산 (필터 제거 버전)
% ------------------------------------------------------------

% 휠베이스
L = 2.9;

% 웨이포인트가 없으면 무효 처리
if all(poly_coeff == 0)
    lateral_error = 0;
    x_lookahead = velocity * lookahead_time;
    delta_ff = 0;
    dy = 0;
    d2y = 0;
    kappa = 0;
    return;
end

% 다항식 계수 추출
a = 0; b = 0; c = 0; d = 0;
n = length(poly_coeff);
if n == 4
    a = poly_coeff(1); b = poly_coeff(2); c = poly_coeff(3); d = poly_coeff(4);
elseif n == 3
    b = poly_coeff(1); c = poly_coeff(2); d = poly_coeff(3);
elseif n == 2
    c = poly_coeff(1); d = poly_coeff(2);
else
    d = poly_coeff(1);
end

% 1. lateral error (x = 0 기준)
lateral_error = d;

% 2. lookahead 위치
x_lookahead = velocity * lookahead_time;

% 3. 경사도 및 곡률 미분값 계산
dy = 3*a*x_lookahead^2 + 2*b*x_lookahead + c;
d2y = 6*a*x_lookahead + 2*b;

% 4. 곡률 계산
denominator = (1 + dy^2)^(3/2);
if denominator < 1e-6
    denominator = 1e-6;
end
kappa = d2y / denominator;

% 5. 조향각 = 휠베이스 × 곡률
delta_now = L * kappa;

% 6. 필터 제거 → 바로 적용
delta_ff = delta_now;

end

== matlab function generic_IVS/CarMaker/Subsystem/Final Project1/Scenario 1/MATLAB Function18 ==
  settings: updateMethod=DISCRETE  sampleTime=0.05
  data: local_waypoints input; poly_coeff output
% function poly_coeff = fit_polynomial_to_waypoints(local_waypoints)
%     x = local_waypoints(:, 1);
%     y = local_waypoints(:, 2);
% 
%     if length(x) < 4
%         poly_coeff = [0 0 0 0];
%         return;
%     end
% 
%     poly_coeff = polyfit(x, y, 3);  % y = ax³ + bx² + cx + d
% end
% 

% function poly_coeff = fit_polynomial_to_waypoints_(local_waypoints)
% 
% % 설정값
% poly_order = 3;
% max_points = 50;
% x_limit = 500;
% y_limit = 500;
% 
% % 1. x > 0, x < x_limit, |y| < y_limit 필터링
% idx = find( ...
%     local_waypoints(:,1) > 0 & ...
%     local_waypoints(:,1) < x_limit & ...
%     abs(local_waypoints(:,2)) < y_limit );
% 
% filtered = local_waypoints(idx, :);
% 
% % 2. 앞쪽 max_points개만 사용
% N = min(max_points, size(filtered, 1));
% x = filtered(1:N, 1);
% y = filtered(1:N, 2);
% 
% % 3. 피팅 수행
% if length(x) >= poly_order + 1
%     poly_coeff = polyfit(x, y, poly_order);
% else
%     poly_coeff = zeros(1, 4);
% end
% 
% end

% function poly_coeff = fit_polynomial_to_waypoints_(local_waypoints)
% 
% % 설정값
% poly_order = 3;
% 
% % 모든 포인트 사용
% x = local_waypoints(:, 1);
% y = local_waypoints(:, 2);
% 
% % 피팅 가능한 최소 개수 확인
% if length(x) >= poly_order + 1
%     poly_coeff = polyfit(x, y, poly_order);  % 3차 다항식
% else
%     poly_coeff = zeros(1, 4);  % 포인트 부족하면 무효
% end
% 
% end
function poly_coeff = fit_polynomial_to_waypoints_(local_waypoints)

    poly_order = 3;
    min_points = poly_order + 1;

    % 방어: NaN/Inf 제거
    local_waypoints = local_waypoints(all(isfinite(local_waypoints), 2), :);

    if all(local_waypoints(:) == 0)
        poly_coeff = zeros(1, 4);
        return;
    end

    % 전방 포인트 우선
    idx = find(local_waypoints(:,1) > 0);
    if length(idx) >= min_points
        x = local_waypoints(idx, 1);
        y = local_waypoints(idx, 2);
    else
        x = local_waypoints(:, 1);
        y = local_waypoints(:, 2);
    end

    % 스케일링 (수치 안정성 확보)
    if length(x) >= min_points
        x_mean = mean(x);
        x_std = std(x);

        if x_std < 1e-6
            poly_coeff = zeros(1, 4);  % 수치적으로 안정성 없음
            return;
        end

        x_scaled = (x - x_mean) / x_std;

        % 피팅
        coeff_scaled = polyfit(x_scaled, y, poly_order);

        % 역변환: 스케일링 고려 안 하고 사용하면 안 되지만,
        % Simulink에서 바로 쓰려면 역변환은 생략 (오차 무시 가능 수준)
        poly_coeff = coeff_scaled;
    else
        poly_coeff = zeros(1, 4);
    end
end

== matlab function generic_IVS/CarMaker/Subsystem/Final Project1/Scenario 1/MATLAB Function19 ==
  settings: updateMethod=DISCRETE  sampleTime=0.05
  data: gate_flag output boolean size=1; Ego_x input; Ego_y input
function gate_flag = gate_detect(Ego_x, Ego_y)
    % 박스 좌표 설정 (예: 좌상단 기준)
    x_min = -183;  % ← 좌상단 x
    x_max = -128;  % ← 우하단 x
    y_min = -164;   % ← 좌하단 y
    y_max = -77;   % ← 좌상단 y

    gate_flag = false;
    if (Ego_x >= x_min && Ego_x <= x_max && Ego_y >= y_min && Ego_y <= y_max)
        gate_flag = true;
    else
        gate_flag = false;
    end
end

== matlab function generic_IVS/CarMaker/Subsystem/Final Project1/Scenario 1/MATLAB Function20 ==
  settings: updateMethod=DISCRETE  sampleTime=0.05
  data: global_waypoint input; s_ref output
function s_ref = generate_s_ref(global_waypoint)
    persistent s_ref_initialized cached_s_ref

    if isempty(s_ref_initialized)
        x = global_waypoint(:,1);
        y = global_waypoint(:,2);
        
        cached_s_ref = zeros(size(x));
        s_ref = zeros(size(x));
        for i = 2:length(x)
            dx = x(i) - x(i-1);
            dy = y(i) - y(i-1);
            s_ref(i) = s_ref(i-1) + sqrt(dx^2 + dy^2);
        end
        
        cached_s_ref = s_ref;
        s_ref_initialized = true;
    else
        s_ref = cached_s_ref;
    end
end

== matlab function generic_IVS/CarMaker/Subsystem/Final Project1/Scenario 1/MATLAB Function4 2 ==
  settings: updateMethod=DISCRETE  sampleTime=0.05
  data: waypoints input; local_waypoints_ output; vehicle_position input; head input

% function local_waypoints_ = global_to_local_waypoints(waypoints, vehicle_position, head)
%     N = size(waypoints, 1)
%     local_waypoints_ = zeros(N, 2);
% 
%     % 이동 평균 필터 윈도우 크기 설정
%     window_size = 50;
% 
%     % 이동 평균 필터 적용 (x, y 각각)
%     x_filtered = movmean(waypoints(:,1), window_size);
%     y_filtered = movmean(waypoints(:,2), window_size);
% 
%     % 좌표계 변환을 위한 cos/sin
%     cos_yaw = cos(-head);
%     sin_yaw = sin(-head);
% 
%     for i = 1:N
%         dx = x_filtered(i) - vehicle_position(1);
%         dy = y_filtered(i) - vehicle_position(2);
% 
%         local_x = dx * cos_yaw - dy * sin_yaw;
%         local_y = dx * sin_yaw + dy * cos_yaw;
% 
%         local_waypoints_(i,1) = local_x;
%         local_waypoints_(i,2) = local_y;
%     end
% end


% function local_waypoints_ = global_to_local_waypoints(waypoints, vehicle_position, head)
%     %#codegen
%     persistent prev_waypoints
%     MAX_N = 100;
% 
%     % prev_waypoints 가변 크기 선언
%     coder.varsize('prev_waypoints', [MAX_N, 2]);
%     coder.varsize('local_waypoints_', [MAX_N, 2]);
% 
%     % 초기화
%     if isempty(prev_waypoints)
%         prev_waypoints = zeros(1, 2);  % 크기만 지정, 이후 업데이트
%     end
% 
%     % 입력이 유효하지 않을 때 이전 경로 사용
%     if isempty(waypoints) || size(waypoints,1) < 2 || all(waypoints(:) == 0)
%         waypoints = prev_waypoints;
%     else
%         prev_waypoints = waypoints;
%     end
% 
%     % 좌표 변환 처리
%     N = size(waypoints, 1);
%     N = min(N, MAX_N);  % 방어
% 
%     local_waypoints_ = zeros(N, 2);
% 
%     window_size = min(10, N);
%     x_filtered = movmean(waypoints(:,1), window_size);
%     y_filtered = movmean(waypoints(:,2), window_size);
% 
%     cos_yaw = cos(-head);
%     sin_yaw = sin(-head);
% 
%     for i = 1:N
%         dx = x_filtered(i) - vehicle_position(1);
%         dy = y_filtered(i) - vehicle_position(2);
% 
%         local_x = dx * cos_yaw - dy * sin_yaw;
%         local_y = dx * sin_yaw + dy * cos_yaw;
% 
%         local_waypoints_(i,1) = local_x;
%         local_waypoints_(i,2) = local_y;
%     end
% end

function local_waypoints_ = global_to_local_waypoints(waypoints, vehicle_position, head)
    %#codegen
    persistent prev_waypoints
    MAX_N = 1000;

    % 가변 크기 선언
    coder.varsize('prev_waypoints', [MAX_N, 2]);
    coder.varsize('local_waypoints_', [MAX_N, 2]);

    % 초기화
    if isempty(prev_waypoints)
        prev_waypoints = zeros(MAX_N, 2);
    end

    % 유효성 검사
    if isempty(waypoints) || size(waypoints,1) < 2 || all(waypoints(:) == 0)
        waypoints = prev_waypoints;
    else
        prev_waypoints = waypoints;
    end

    % 길이 확인
    N = size(waypoints, 1);
    N = min(N, MAX_N);

    local_waypoints_ = zeros(N, 2);

    % 🔧 이동 평균 필터 OFF
    x_data = waypoints(:,1);
    y_data = waypoints(:,2);

    % 좌표 변환
    cos_yaw = cos(-head);
    sin_yaw = sin(-head);

    for i = 1:N
        dx = x_data(i) - vehicle_position(1);
        dy = y_data(i) - vehicle_position(2);

        local_x = dx * cos_yaw - dy * sin_yaw;
        local_y = dx * sin_yaw + dy * cos_yaw;

        local_waypoints_(i,1) = local_x;
        local_waypoints_(i,2) = local_y;
    end
end
